simulink model "Sistema"  (R2016a)
settings: Solver=VariableStepAuto  StartTime=0.0  StopTime=10.0  RelTol=1e-3
undefined symbols (not defined in the file): Bm, Ea, Jm, Kb, Kt, La, Ra
settings Model: Creator=Marcelo  LastModifiedBy=Marcelo

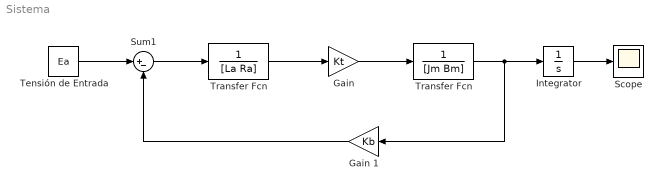
== system Sistema ==
  Gain : Gain  Gain=Kt
  Gain 1 : Gain  Gain=Kb
  Integrator : Integrator
  Scope : Scope
  Sum1 : Sum  Inputs=|+-
  Tensión de Entrada : Constant  Value=Ea
  Transfer Fcn : TransferFcn  Denominator=[La Ra]
  "Transfer Fcn " : TransferFcn  Denominator=[Jm Bm]
  wires:
  Sum1/1 -> Transfer Fcn/1
  Tensión de Entrada/1 -> Sum1/1
  Gain 1/1 -> Sum1/2
  Transfer Fcn/1 -> Gain/1
  "Transfer Fcn "/1 -> Integrator/1, Gain 1/1
  Integrator/1 -> Scope/1
  Gain/1 -> "Transfer Fcn "/1
